simulink library "MonoDetector"  (R2022b)
settings: Solver=VariableStepAuto  StartTime=0.0  StopTime=10.0  RelTol=1e-3
undefined symbols (not defined in the file or in its folder): Row
libraries: TuneVar x14, TOP x12, StateVar x3, HandyTextFile x2, CapturedConstLib x2, FeaturePath x1, AudioStats x1, simulink x1, PoolIir x1
settings Model: Creator=ud1041536  LastModifiedBy=sc48041
settings SolverCC: AlgebraicLoopSolver=TrustRegion
settings DebuggingCC: UnconnectedInputMsg=warning  UnconnectedOutputMsg=warning  UnconnectedLineMsg=warning  SFMachineParentedDataDiag=warning  ArithmeticOperatorsInVariantConditions=warning
settings ModelReferenceCC: EnableRefExpFcnMdlSchedulingChecks=on
settings SFSimCC: CustomCodeUndefinedFunction=UseInterfaceOnly

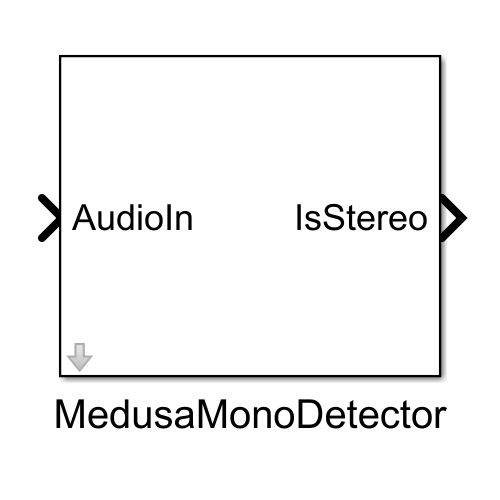
[thumbnail: Simulink's stored preview of the top-level diagram]
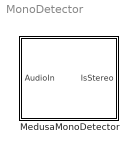
== system MonoDetector ==
  MedusaMonoDetector : Subsystem  mask(Mono Detector){Config=[]}
      mask prompts: Config "MedusaMonoDetectorConfig"
      mask help:
      | This block detects if given stereo input (L, R) is stereo. The output isStereo is used to enable/disable Spatial Unmasker in Medusa system. When the block is put to passthrough by tuning, the default output is set to 'true'.
      |
      | Configuration struct needs to define the below fields with the exact names which are used inside the block.
      |
      | decimationFactor: decimation factor
      | maxZeroLevelCount: maximum number of zero signals in a row before reset
      | hpfOrder: order of highpass filter
      | maxNumStages: maximum of sos for both L and R highpass filter
      | numChannels: number of channels
      |
      | For more information and sample generation of config struct, please see 'Help'.
      mask init:
      | blkh=gcbh;
      | Config=BTConfig.Assert(blkh,Config);
      | 
      | Config.Validate();
      mask Help:
      | Model that uses Mono Detector block need to call MonoDetectorInit(config) to generate <i>MonoDetectorConfigStruct</i> and <i>MonoDetectorTunable</i> bus object in base workspace.
      | 
      | <b>Sample usage:</b>
      | 
      | MedusaConfig = generateMedusaConfig(auto_gen_sys_defs);
      | MonoDetectorInit(MedusaConfig);
      | or
      | DefaultMedusaConfig = generateMedusaConfig();
      | MonoDetectorInit(DefaultMedusaConfig);

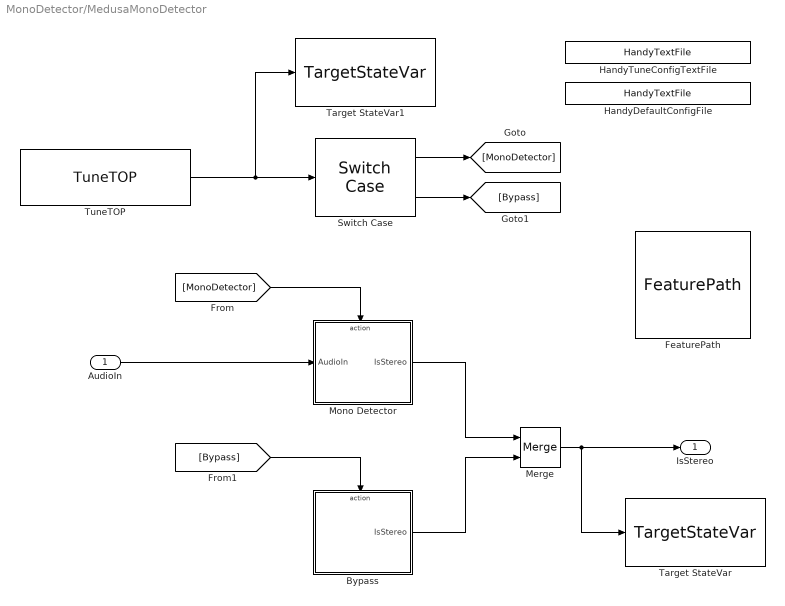
== system MonoDetector/MedusaMonoDetector ==
  AudioIn : Inport
  Bypass : Subsystem
  FeaturePath : FeaturePath/FeaturePath  FeatureName=MonoDetector  IsGroup=off  GroupNumber=-1  IsModule=off  TriggerInit=[680 129 795 236]
      settings: SourceProductName=Bose Talaria
  HandyDefaultConfigFile : HandyTextFile/HandyTextFile  TemplateSource=Config  FileSuffix=Init  OpenDialogOnLoad=off  UseThisBlockName=off  AddGrandParentNamePrefix=off  TheDefaultText=|  ShowInLibBrowser=on
      | % $(FILENAME) Setup model parameters for each "Init" callback (e.g. update diagram)
      | sample_rate_in_hertz = 44100;
      | frame_size = 32;
      | sysin_channel_count = 2;
      settings: SourceProductName=Bose Talaria
  HandyTuneConfigTextFile : HandyTextFile/HandyTextFile  TemplateSource=TuneConfig  FileSuffix=Init  OpenDialogOnLoad=off  UseThisBlockName=off  AddGrandParentNamePrefix=off  TheDefaultText=|  ShowInLibBrowser=on
      | % $(FILENAME) Setup model parameters for each "Init" callback (e.g. update diagram)
      | sample_rate_in_hertz = 44100;
      | frame_size = 32;
      | sysin_channel_count = 2;
      settings: SourceProductName=Bose Talaria
  Merge : Merge
  Mono Detector : Subsystem
  Switch Case : SwitchCase
  Target StateVar : StateVar/TargetStateVar  TriggerInit=[670 396 810 464]  TspName=IsStereo  StateName=IsStereo  UseSameName=on  IfdefMacro=[]
      settings: SourceProductName=Bose Talaria
  Target StateVar1 : StateVar/TargetStateVar  TriggerInit=[340 131 480 199]  TspName=IsActive  StateName=IsActive  UseSameName=on  IfdefMacro=[]
      settings: SourceProductName=Bose Talaria
  TuneTOP : TuneVar/TuneTOP  TriggerInit=[65 47 235 103]  TopName=Enable  TuneName=Enable  DataTypeOut=int32  TunabilityNumber=1  MinValue=[]  MaxValue=[]  BankNumber=0  PreOverlay=false  PostOverlay=false  UseSameName=on  MaskValue=Config.TuneDefaults.Enable
      settings: SourceProductName=Bose Talaria
  IsStereo : Outport  VectorParamsAs1DForOutWhenUnconnected=off
  wires:
  Merge/1 -> Target StateVar/1, IsStereo/1
  Switch Case/1 -> [MonoDetector]
  TuneTOP/1 -> Switch Case/1, Target StateVar1/1
  AudioIn/1 -> Mono Detector/1(AudioIn)
  Bypass/1(IsStereo) -> Merge/2
  Switch Case/2 -> [Bypass]
  Mono Detector/1(IsStereo) -> Merge/1
  [Bypass] -> Bypass/Action
  [MonoDetector] -> Mono Detector/Action

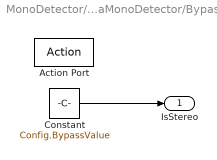
== system MonoDetector/MedusaMonoDetector/Bypass ==
  Action Port : ActionPort  ActionPortLabel=default: { }
  Constant : Constant  Value=Config.BypassValue  OutDataTypeStr=uint32
  IsStereo : Outport  VectorParamsAs1DForOutWhenUnconnected=off
  wires:
  Constant/1 -> IsStereo/1

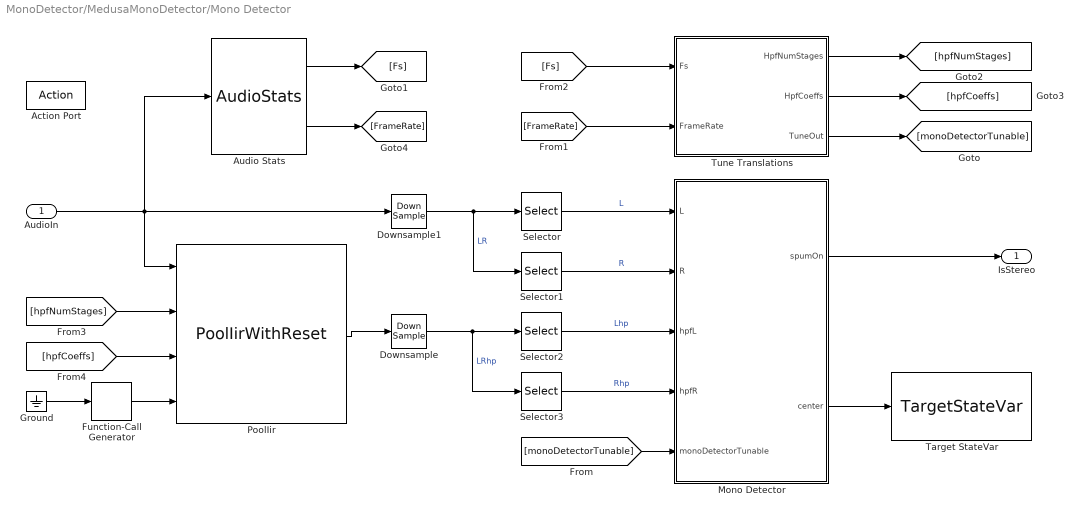
== system MonoDetector/MedusaMonoDetector/Mono Detector ==
  AudioIn : Inport  OutDataTypeStr=single
  Action Port : ActionPort  ActionPortLabel=case: { }
  Audio Stats : AudioStats/AudioStats  DoSampleRate=on  TypeSampleRate=double  DoCallRate=on  TypeCallRate=double  DoFrameSize=off  TypeFrameSize=Inherit: auto  DoChannelCount=off  TypeChannelCount=Inherit: auto  DoTaskRateFactor=off  TypeTaskRateFactor=Inherit: auto  MacroNameRoot=AUDIO  MacroNameRootEval='AUDIO'  IsMacroNameEval=off  MacroSampleRate=off  MacroCallRate=off  MacroFrameSize=off  MacroChannelCount=off  MacroTaskRateFactor=off  MacroTaskId=off  ValidateSampleRate=off  ValueSampleRate=[]  ValidateCallRate=off  ValueCallRate=[]  ValidateFrameSize=off  ValueFrameSize=[]  ValidateChannelCount=off  ValueChannelCount=[]  ValidateTaskRateFactor=off  ValueTaskRateFactor=[]
      settings: SourceProductName=Bose Talaria
  Downsample : DownSample  N=Config.DownSamplingFactor
  Downsample1 : DownSample  N=Config.DownSamplingFactor
  Function-Call Generator : simulink/Ports & Subsystems/Function-Call Generator  sample_time=1  numberOfIterations=1  DisallowWideOutput=off  ShowEnablePort=on
  Ground : Ground
  Mono Detector : MATLAB Function  TreatAsAtomicUnit=on  mask{maxZeroLevelCount=Config.MaxZeroLevelCount}
  PoolIir : PoolIir/PoolIirWithReset  Config=Config.Hpf
  Selector : Selector  InputPortWidth=2  IndexOptions=Index vector (dialog)  Indices=1  OutputSizes=1
  Selector1 : Selector  InputPortWidth=2  IndexOptions=Index vector (dialog)  Indices=2  OutputSizes=1
  Selector2 : Selector  InputPortWidth=2  IndexOptions=Index vector (dialog)  Indices=1  OutputSizes=1
  Selector3 : Selector  InputPortWidth=2  IndexOptions=Index vector (dialog)  Indices=2  OutputSizes=1
  Target StateVar : StateVar/TargetStateVar  TriggerInit=[875 1951 1015 2019]  TspName=LevelCenter  StateName=LevelCenter  UseSameName=on  IfdefMacro=[]
      settings: SourceProductName=Bose Talaria
  Tune Translations : Subsystem
  IsStereo : Outport  VectorParamsAs1DForOutWhenUnconnected=off
  wires:
  Downsample1/1 -> Selector1/1, Selector/1  "LR"
  Mono Detector/2(center) -> Target StateVar/1
  Downsample/1 -> Selector3/1, Selector2/1  "LRhp"
  Selector/1 -> Mono Detector/1(L)  "L"
  [hpfCoeffs] -> PoolIir/3
  PoolIir/1 -> Downsample/1
  [hpfNumStages] -> PoolIir/2
  Selector1/1 -> Mono Detector/2(R)  "R"
  Audio Stats/1 -> [Fs]
  Mono Detector/1(spumOn) -> IsStereo/1
  [monoDetectorTunable] -> Mono Detector/5(monoDetectorTunable)
  Selector2/1 -> Mono Detector/3(hpfL)  "Lhp"
  Selector3/1 -> Mono Detector/4(hpfR)  "Rhp"
  AudioIn/1 -> PoolIir/1, Downsample1/1, Audio Stats/1
  Audio Stats/2 -> [FrameRate]
  [Fs] -> Tune Translations/1(Fs)
  [FrameRate] -> Tune Translations/2(FrameRate)
  Tune Translations/3(TuneOut) -> [monoDetectorTunable]
  Tune Translations/2(HpfCoeffs) -> [hpfCoeffs]
  Tune Translations/1(HpfNumStages) -> [hpfNumStages]
  Ground/1 -> Function-Call Generator/1
  Function-Call Generator/1 -> PoolIir/4

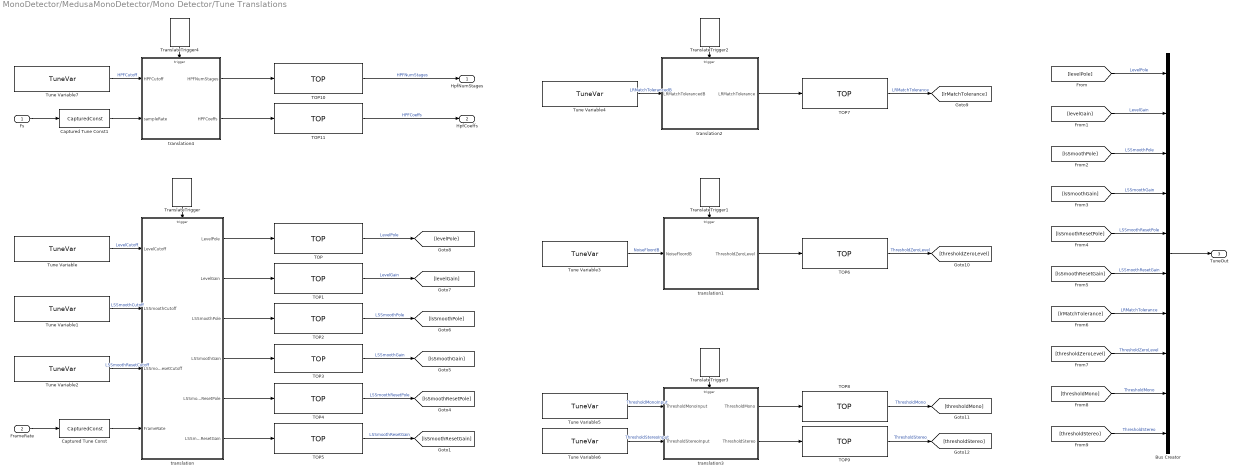
== system MonoDetector/MedusaMonoDetector/Mono Detector/Tune Translations ==
  Fs : Inport
  FrameRate : Inport  Port=2
  Bus Creator : BusCreator  Inputs=10  OutDataTypeStr=Bus: MonoDetectorTunable
      settings: InheritFromInputs=off
  Captured Tune Const : CapturedConstLib/CapturedConst  TriggerInit=[-1540 1092 -1440 1128]  Role=Automatic
      settings: SourceProductName=Bose Talaria
  Captured Tune Const1 : CapturedConstLib/CapturedConst  TriggerInit=[-1540 472 -1440 508]  Role=Automatic
      settings: SourceProductName=Bose Talaria
  TOP : TOP/TOP  TriggerInit=[-1110 700 -935 760]  TopName=LevelPole  DataTypeOut=single  BankNumber=0  PreOverlay=false  PostOverlay=false  Role=Automatic
      settings: SourceProductName=Bose Talaria
  TOP1 : TOP/TOP  TriggerInit=[-1110 780 -935 840]  TopName=LevelGain  DataTypeOut=single  BankNumber=0  PreOverlay=false  PostOverlay=false  Role=Automatic
      settings: SourceProductName=Bose Talaria
  TOP10 : TOP/TOP  TriggerInit=[-1110 380 -935 440]  TopName=HPFNumStages  DataTypeOut=uint32  BankNumber=0  PreOverlay=false  PostOverlay=false  Role=Automatic
      settings: SourceProductName=Bose Talaria
  TOP11 : TOP/TOP  TriggerInit=[-1110 460 -935 520]  TopName=HPFCoeffs  DataTypeOut=single  BankNumber=0  PreOverlay=false  PostOverlay=false  Role=Automatic
      settings: SourceProductName=Bose Talaria
  TOP2 : TOP/TOP  TriggerInit=[-1110 860 -935 920]  TopName=LSSmoothPole  DataTypeOut=single  BankNumber=0  PreOverlay=false  PostOverlay=false  Role=Automatic
      settings: SourceProductName=Bose Talaria
  TOP3 : TOP/TOP  TriggerInit=[-1110 942 -935 998]  TopName=LSSmoothGain  DataTypeOut=single  BankNumber=0  PreOverlay=false  PostOverlay=false  Role=Automatic
      settings: SourceProductName=Bose Talaria
  TOP4 : TOP/TOP  TriggerInit=[-1110 1020 -935 1080]  TopName=LSSmoothResetPole  DataTypeOut=single  BankNumber=0  PreOverlay=false  PostOverlay=false  Role=Automatic
      settings: SourceProductName=Bose Talaria
  TOP5 : TOP/TOP  TriggerInit=[-1110 1100 -935 1160]  TopName=LSSmoothResetGain  DataTypeOut=single  BankNumber=0  PreOverlay=false  PostOverlay=false  Role=Automatic
      settings: SourceProductName=Bose Talaria
  TOP6 : TOP/TOP  TriggerInit=[-55 730 115 790]  TopName=ThresholdZeroLevel  DataTypeOut=single  BankNumber=0  PreOverlay=false  PostOverlay=false  Role=Automatic
      settings: SourceProductName=Bose Talaria
  TOP7 : TOP/TOP  TriggerInit=[-55 410 115 470]  TopName=LRMatchTolerance  DataTypeOut=single  BankNumber=0  PreOverlay=false  PostOverlay=false  Role=Automatic
      settings: SourceProductName=Bose Talaria
  TOP8 : TOP/TOP  TriggerInit=[-55 1035 115 1095]  TopName=ThresholdMono  DataTypeOut=single  BankNumber=0  PreOverlay=false  PostOverlay=false  Role=Automatic
      settings: SourceProductName=Bose Talaria
  TOP9 : TOP/TOP  TriggerInit=[-55 1105 115 1165]  TopName=ThresholdStereo  DataTypeOut=single  BankNumber=0  PreOverlay=false  PostOverlay=false  Role=Automatic
      settings: SourceProductName=Bose Talaria
  TranslateTrigger : TuneVar/TranslateTrigger  TriggerInit=[-1314 610 -1276 665]
      settings: SourceProductName=Bose Talaria
  TranslateTrigger1 : TuneVar/TranslateTrigger  TriggerInit=[-259 610 -221 665]
      settings: SourceProductName=Bose Talaria
  TranslateTrigger2 : TuneVar/TranslateTrigger  TriggerInit=[-259 290 -221 345]
      settings: SourceProductName=Bose Talaria
  TranslateTrigger3 : TuneVar/TranslateTrigger  TriggerInit=[-259 950 -221 1005]
      settings: SourceProductName=Bose Talaria
  TranslateTrigger4 : TuneVar/TranslateTrigger  TriggerInit=[-1319 290 -1281 345]
      settings: SourceProductName=Bose Talaria
  Tune Variable : TuneVar/TuneVar  TuneName=LevelCutoff  SpecifyMaxSize=off  VariableDim=1 (Row)  MaxSize=[1 1]  TunabilityNumber=1  MinValue=[]  MaxValue=[]  TriggerInit=[-1630 725 -1440 775]  MaskValue=Config.TuneDefaults.LevelCutoff
      settings: SourceProductName=Bose Talaria
  Tune Variable1 : TuneVar/TuneVar  TuneName=LSSmoothCutoff  SpecifyMaxSize=off  VariableDim=1 (Row)  MaxSize=[1 1]  TunabilityNumber=1  MinValue=[]  MaxValue=[]  TriggerInit=[-1630 845 -1440 895]  MaskValue=Config.TuneDefaults.LSSmoothCutoff
      settings: SourceProductName=Bose Talaria
  Tune Variable2 : TuneVar/TuneVar  TuneName=LSSmoothResetCutoff  SpecifyMaxSize=off  VariableDim=1 (Row)  MaxSize=[1 1]  TunabilityNumber=1  MinValue=[]  MaxValue=[]  TriggerInit=[-1630 965 -1440 1015]  MaskValue=Config.TuneDefaults.LSSmoothResetCutoff
      settings: SourceProductName=Bose Talaria
  Tune Variable3 : TuneVar/TuneVar  TuneName=NoiseFloordB  SpecifyMaxSize=off  VariableDim=1 (Row)  MaxSize=[1 1]  TunabilityNumber=1  MinValue=[]  MaxValue=[]  TriggerInit=[-575 735 -405 785]  MaskValue=Config.TuneDefaults.NoiseFloordB
      settings: SourceProductName=Bose Talaria
  Tune Variable4 : TuneVar/TuneVar  TuneName=LRMatchTolerancedB  SpecifyMaxSize=off  VariableDim=1 (Row)  MaxSize=[1 1]  TunabilityNumber=1  MinValue=[]  MaxValue=[]  TriggerInit=[-575 415 -385 465]  MaskValue=Config.TuneDefaults.LRMatchTolerancedB
      settings: SourceProductName=Bose Talaria
  Tune Variable5 : TuneVar/TuneVar  TuneName=ThresholdMonoInput  SpecifyMaxSize=off  VariableDim=1 (Row)  MaxSize=[1 1]  TunabilityNumber=1  MinValue=[]  MaxValue=[]  TriggerInit=[-575 1040 -405 1090]  MaskValue=Config.TuneDefaults.ThresholdMonoInput
      settings: SourceProductName=Bose Talaria
  Tune Variable6 : TuneVar/TuneVar  TuneName=ThresholdStereoInput  SpecifyMaxSize=off  VariableDim=1 (Row)  MaxSize=[1 1]  TunabilityNumber=1  MinValue=[]  MaxValue=[]  TriggerInit=[-575 1110 -405 1160]  MaskValue=Config.TuneDefaults.ThresholdStereoInput
      settings: SourceProductName=Bose Talaria
  Tune Variable7 : TuneVar/TuneVar  TuneName=HPFCutoff  SpecifyMaxSize=off  VariableDim=1 (Row)  MaxSize=[1 1]  TunabilityNumber=1  MinValue=[]  MaxValue=[]  TriggerInit=[-1630 385 -1440 435]  MaskValue=Config.TuneDefaults.HPFCutoff
      settings: SourceProductName=Bose Talaria
  translation : MATLAB Function  TreatAsAtomicUnit=on
  translation1 : MATLAB Function  TreatAsAtomicUnit=on
  translation2 : MATLAB Function  TreatAsAtomicUnit=on
  translation3 : MATLAB Function  TreatAsAtomicUnit=on
  translation4 : MATLAB Function  TreatAsAtomicUnit=on  mask{numChannels=Config.NumInputChannels, maxNumStages=Config.Hpf.MaxNumStages}
  HpfNumStages : Outport
  HpfCoeffs : Outport  Port=2
  TuneOut : Outport  Port=3
  wires:
  Tune Variable1/1 -> translation/2(LSSmoothCutoff)  "LSSmoothCutoff"
  Tune Variable6/1 -> translation3/2(ThresholdStereoInput)  "ThresholdStereoInput"
  translation3/1(ThresholdMono) -> TOP8/1
  [thresholdMono] -> Bus Creator/9  "ThresholdMono"
  [lsSmoothResetGain] -> Bus Creator/6  "LSSmoothResetGain"
  Tune Variable/1 -> translation/1(LevelCutoff)  "LevelCutoff"
  [lsSmoothResetPole] -> Bus Creator/5  "LSSmoothResetPole"
  Tune Variable4/1 -> translation2/1(LRMatchTolerancedB)  "LRMatchTolerancedB"
  translation/3(LSSmoothPole) -> TOP2/1
  translation4/2(HPFCoeffs) -> TOP11/1
  translation/5(LSSmoothResetPole) -> TOP4/1
  FrameRate/1 -> Captured Tune Const/1
  TOP10/1 -> HpfNumStages/1  "HPFNumStages"
  [thresholdZeroLevel] -> Bus Creator/8  "ThresholdZeroLevel"
  Captured Tune Const/1 -> translation/4(FrameRate)
  TranslateTrigger2/1 -> translation2/Trigger
  translation3/2(ThresholdStereo) -> TOP9/1
  TranslateTrigger3/1 -> translation3/Trigger
  [thresholdStereo] -> Bus Creator/10  "ThresholdStereo"
  TranslateTrigger1/1 -> translation1/Trigger
  Tune Variable5/1 -> translation3/1(ThresholdMonoInput)  "ThresholdMonoInput"
  Tune Variable7/1 -> translation4/1(HPFCutoff)  "HPFCutoff"
  translation2/1(LRMatchTolerance) -> TOP7/1
  Fs/1 -> Captured Tune Const1/1
  translation/4(LSSmoothGain) -> TOP3/1
  Bus Creator/1 -> TuneOut/1
  [lrMatchTolerance] -> Bus Creator/7  "LRMatchTolerance"
  TranslateTrigger4/1 -> translation4/Trigger
  TranslateTrigger/1 -> translation/Trigger
  [levelPole] -> Bus Creator/1  "LevelPole"
  translation1/1(ThresholdZeroLevel) -> TOP6/1
  TOP11/1 -> HpfCoeffs/1  "HPFCoeffs"
  [levelGain] -> Bus Creator/2  "LevelGain"
  [lsSmoothGain] -> Bus Creator/4  "LSSmoothGain"
  Captured Tune Const1/1 -> translation4/2(sampleRate)
  Tune Variable3/1 -> translation1/1(NoiseFloordB)  "NoiseFloordB"
  translation/6(LSSmoothResetGain) -> TOP5/1
  translation4/1(HPFNumStages) -> TOP10/1
  translation/1(LevelPole) -> TOP/1
  Tune Variable2/1 -> translation/3(LSSmoothResetCutoff)  "LSSmoothResetCutoff"
  translation/2(LevelGain) -> TOP1/1
  [lsSmoothPole] -> Bus Creator/3  "LSSmoothPole"
  TOP5/1 -> [lsSmoothResetGain]  "LSSmoothResetGain"
  TOP4/1 -> [lsSmoothResetPole]  "LSSmoothResetPole"
  TOP3/1 -> [lsSmoothGain]  "LSSmoothGain"
  TOP2/1 -> [lsSmoothPole]  "LSSmoothPole"
  TOP1/1 -> [levelGain]  "LevelGain"
  TOP/1 -> [levelPole]  "LevelPole"
  TOP7/1 -> [lrMatchTolerance]  "LRMatchTolerance"
  TOP6/1 -> [thresholdZeroLevel]  "ThresholdZeroLevel"
  TOP8/1 -> [thresholdMono]  "ThresholdMono"
  TOP9/1 -> [thresholdStereo]  "ThresholdStereo"

== matlab function MonoDetector/MedusaMonoDetector/Mono Detector/Tune Translations/translation1 ==
  data: ThresholdZeroLevel output; NoiseFloordB input
  events: trigger input FUNCTION_CALL_EVENT
function ThresholdZeroLevel  = fcn(NoiseFloordB)
% thresh = 2 * undb20(noiseFloordB)
ThresholdZeroLevel = 2 * (10 ^ (NoiseFloordB.Value / 20));

== matlab function MonoDetector/MedusaMonoDetector/Mono Detector/Mono Detector ==
  data: L input; spumOn output; R input; hpfL input; hpfR input; center output; monoDetectorTunable input; maxZeroLevelCount parameter
function [spumOn, center]  = monoDetect(L, R, hpfL, hpfR, ...
                                monoDetectorTunable, maxZeroLevelCount)
%#codegen

persistent zeroLevelCount;
persistent Llevel;
persistent Rlevel;
persistent smoothedSumOfEnergies;
persistent smoothedEnergyOfSum;
persistent levelCenter;
persistent lastSpumOn; % basically isStereo, since we turn on SPUM if input is stereo

if isempty(zeroLevelCount); zeroLevelCount = 0; end
if isempty(Llevel); Llevel = single(0); end
if isempty(Rlevel); Rlevel = single(0); end
if isempty(smoothedSumOfEnergies); smoothedSumOfEnergies = single(0); end
if isempty(smoothedEnergyOfSum); smoothedEnergyOfSum = single(0); end
if isempty(levelCenter); levelCenter = single(0); end
if isempty(lastSpumOn); lastSpumOn = true; end

absLeft = abs(L);
absRight = abs(R);

% Recursive averaging
a1 = monoDetectorTunable.levelPole;
b0 = monoDetectorTunable.levelGain;
Llevel = Llevel * a1 +  absLeft * b0;
Rlevel = Rlevel * a1 +  absRight * b0;

% Compute saturated signals from predetermined miss-match tolerance
LlevelSat = min(Llevel, Rlevel*monoDetectorTunable.leftRightMatchTolerance);
RlevelSat = min(Rlevel, Llevel*monoDetectorTunable.leftRightMatchTolerance);

% Compute mono content variables
curL = hpfL * RlevelSat;
curR = hpfR * LlevelSat;
sumOfEnergies = curL^2 + curR^2; % tgtX2
energyOfSum = 0.5*(curL + curR)^2; % tgtX2Center

% Check if signal has been low for awhile
if (absLeft + absRight) < monoDetectorTunable.thresholdZeroLevel
    zeroLevelCount = zeroLevelCount + 1;
else 
    zeroLevelCount = 0;
end

% Pole selection (determine LPF coefficient) for least square smoothing
% If the signal level is very low (or zero) for awhile, rest params and 
% select correct poles so that we don't miss fast changes in input
if zeroLevelCount > maxZeroLevelCount
    sumOfEnergies = single(0);
    energyOfSum = single(0);
    smoothedSumOfEnergies = single(0);
    smoothedEnergyOfSum = single(0);
    lsPole = monoDetectorTunable.lsSmoothResetPole;
    lsGain = monoDetectorTunable.lsSmoothResetGain;
    zeroLevelCount = maxZeroLevelCount + 1;
else
    lsPole = monoDetectorTunable.lsSmoothPole;
    lsGain = monoDetectorTunable.lsSmoothGain;
end

% Least square smoothing 
smoothedSumOfEnergies = lsPole * smoothedSumOfEnergies + lsGain * sumOfEnergies;
smoothedEnergyOfSum = lsPole * smoothedEnergyOfSum + lsGain * energyOfSum;

% Compute measure of center (or mono) level
levelCenter = smoothedEnergyOfSum/(smoothedSumOfEnergies + single(eps));

% Determine if input is stereo and turn SPUM on/off accordingly
% stereo case 1: was stereo last time (SPUM on) and this mono level < mono threhold
% stereo case 2: was mono last time (SPUM off) and this mono level < stereo threshold
lastSpumOn = (lastSpumOn && (levelCenter < monoDetectorTunable.thresholdMono)) ...
    || (~lastSpumOn && (levelCenter <= monoDetectorTunable.thresholdStereo));

spumOn = uint32(lastSpumOn);% equivalent to isStereo

center = levelCenter;

end

== matlab function MonoDetector/MedusaMonoDetector/Mono Detector/Tune Translations/translation2 ==
  data: LRMatchTolerance output; LRMatchTolerancedB input
  events: trigger input FUNCTION_CALL_EVENT
function LRMatchTolerance  = fcn(LRMatchTolerancedB)

if (LRMatchTolerancedB.Value < 0 || LRMatchTolerancedB.Value > 0.5)
    TranslateError('Invalid tolerance for left right match');
    LRMatchTolerance = 0;
else
    LRMatchTolerance = 10 ^ (LRMatchTolerancedB.Value / 20);
end

== matlab function MonoDetector/MedusaMonoDetector/Mono Detector/Tune Translations/translation3 ==
  data: ThresholdMono output; ThresholdMonoInput input; ThresholdStereoInput input; ThresholdStereo output
  events: trigger input FUNCTION_CALL_EVENT
function [ThresholdMono, ThresholdStereo] = fcn(ThresholdMonoInput, ThresholdStereoInput)
% The exponent 1/64 is carried over from AR and old bdsp implementation.
% This is designed by Chris Cheng to make the gap between two thresholds
% as small as possible, because in theory they should be almost identical.
% Removing this would still work in theory with a slight change in the 
% output. However as we verify the block against PREQ Simulink model, this
% translation is retained to get a complete match in performance.

if ThresholdMonoInput.Value <= ThresholdStereoInput.Value
    TranslateError('Threshold for mono should be higher than that for stereo');
    ThresholdMono = 0;
    ThresholdStereo = 0;
elseif (ThresholdMonoInput.Value >= 1) || (ThresholdStereoInput.Value >= 1)
    TranslateError('Threshold values for mono and stereo should be less than 1.0');
    ThresholdMono = 0;
    ThresholdStereo = 0;
else
    ThresholdMono = ThresholdMonoInput.Value ^ (1/64);
    ThresholdStereo = ThresholdStereoInput.Value ^ (1/64);
end

== matlab function MonoDetector/MedusaMonoDetector/Mono Detector/Tune Translations/translation4 ==
  data: HPFNumStages output; HPFCutoff input; sampleRate input; HPFCoeffs output; numChannels parameter; maxNumStages parameter
  events: trigger input FUNCTION_CALL_EVENT
function [HPFNumStages, HPFCoeffs] = fcn(HPFCutoff, sampleRate, numChannels, maxNumStages)
%#codegen
%[Param:numChannels]
%[Param:maxNumStages]

% Calculation is fixed for a second order high pass butterworth, i.e. this 
% translation will not work anymore if the filter order/design is changed. 
% Code for computing hpf is taken from AR model.
% More generic implementation is also included below. In this case of 2nd 
% order filter, we get better precision by getting the one-stage sos 
% directly from the transfer function.

% hpfOrder = configStruct.hpfOrder;
% normFreq = 2 * HPFCutoff.Value / sampleRate;
% [Z, P, K] = butter_for_code_gen(hpfOrder, hpfOrder, normFreq, 'high');
% sos = zp2sos_for_code_gen(Z, P, K);

w = 2 * pi* HPFCutoff.Value / sampleRate;
sqrt2 = sqrt(2);
sinw = sin(w);
cosw = cos(w);

if (HPFCutoff.Value <= 0) || (HPFCutoff.Value > sampleRate/2)
    TranslateError('Highpass filter cutoff is out of range; should be in (0, %d)',sampleRate/2);
    b = single([1 0 0]);
    a = single([1 0 0]);
else
    denom = (sqrt2 + sinw);
    a1 = -2 * sqrt2 * cosw / denom;
    a2 = (sqrt2 - sinw) / denom;
    a = single([1 a1 a2]);
    b = single([1 -2 1] * (1-a1+a2) / 4);
end
sos = [b,a];

numStages = size(sos, 1) * ones(1, numChannels);
rawSOS = repmat(sos, numChannels, 1);

[HPFNumStages, HPFCoeffs] = pooliirTranslation(rawSOS, numStages, maxNumStages);

end


function [PoolNumStages, PoolCoeffs] = pooliirTranslation(rawSOS, numStages, maxNumStages)
% Function to format sos into pooliir. Taken from Translation block
% inside pooliir library block.

RawSOS = rawSOS;
NumStages = int32(numStages);
NumChannels = length(NumStages);

MaxNumStages = maxNumStages; 
PoolNumStages = int32(zeros(NumChannels,1));
PoolCoeffs = double(zeros(MaxNumStages * 4 + NumChannels,1));
ChannelCoeffs = zeros(MaxNumStages * 4 + 1,1);
ChannelSOS = double(zeros(MaxNumStages, 6));
SOSIndex = int32(0);

for i = 1:NumChannels
    
    ChannelNumStages = NumStages(i);   % Size of current SOS
    assert(ChannelNumStages <= MaxNumStages);
    
    ChannelSOS(1:ChannelNumStages,:) = RawSOS(SOSIndex+(1:ChannelNumStages),:);
    SOSIndex = SOSIndex + ChannelNumStages;

    if size(ChannelSOS,2) ~= 6
        TranslateError('SOS matrix must have 6 columns');
    end
    % decompose SOS
   
    ts = 1:4:4*ChannelNumStages;
    ChannelCoeffs(1,1) = prod(ChannelSOS(1:ChannelNumStages,1));        % b0
    
    % the remaining coeffs are compacted forms of the biquads
    ChannelCoeffs(1+ts,1) = ChannelSOS(1:ChannelNumStages,6);           % a2
    ChannelCoeffs(2+ts,1) = ChannelSOS(1:ChannelNumStages,5);           % a1
    if( ChannelSOS(:,1) == 0 )
    ChannelCoeffs(3+ts,1) = 0;                 % b2/b0
    ChannelCoeffs(4+ts,1) = 0;                 % b1/b0
    else
    ChannelCoeffs(3+ts,1) = ...
        ChannelSOS(1:ChannelNumStages,3)./ ...
        ChannelSOS(1:ChannelNumStages,1);  % b2/b0
    ChannelCoeffs(4+ts,1) = ...
        ChannelSOS(1:ChannelNumStages,2)./ ...
        ChannelSOS(1:ChannelNumStages,1);  % b1/b0
    end
    
    % length of Current Channel Coeffs
    ChannelCoeffsLength = 1+4*ChannelNumStages;
    
    % Offset into coefficient array for the current channel
    offset = (i-1)+4*sum(PoolNumStages(1:i-1));
    
    % Verify that the SOS does not violate the maximum number of stages
    % allocated for the pool
    PoolNumStages(i) = int32(ChannelNumStages);
    if sum(PoolNumStages) > MaxNumStages
        TranslateError('Too many second order sections');
    end

    % Store the coefficients
    PoolCoeffs(offset+(1:ChannelCoeffsLength)) = double(ChannelCoeffs(1:ChannelCoeffsLength));   
end
end

== matlab function MonoDetector/MedusaMonoDetector/Mono Detector/Tune Translations/translation ==
  data: LevelPole output; LevelCutoff input; LevelGain output; LSSmoothCutoff input; LSSmoothResetCutoff input; LSSmoothPole output; LSSmoothGain output; LSSmoothResetPole output; LSSmoothResetGain output; FrameRate input
  events: trigger input FUNCTION_CALL_EVENT
function [LevelPole, LevelGain, LSSmoothPole, LSSmoothGain, ...
    LSSmoothResetPole, LSSmoothResetGain] = fcn(LevelCutoff, ...
    LSSmoothCutoff, LSSmoothResetCutoff, FrameRate)

% Cutoff is the inverse of time constant in Hz. So this function
% basically converts reciprocal of time constant to first order iir
% filter coefficient.
% Reference: https://bosecorp.sharepoint.com/sites/ASD3/DSPTeam/Shared%20Documents/DSP_Topics/Comparison%20of%20time%20constant%20conversion%20methods.docx

error = false;
if LevelCutoff.Value <= LSSmoothCutoff.Value
    TranslateError('Least square smoother should smooth more than level smoother');
    error = true;
elseif LSSmoothResetCutoff.Value <= LSSmoothCutoff.Value
    TranslateError('Least square smoother for reset should smooth less than that for normal mode');
    error = true;
end

if (~error)
    wn = 2 * pi * LevelCutoff.Value / FrameRate;
    LevelPole = (1 - sin(wn)) ./ cos(wn);
    LevelGain = 1 - LevelPole;

    wn = 2 * pi * LSSmoothCutoff.Value / FrameRate;
    LSSmoothPole = (1 - sin(wn)) ./ cos(wn);
    LSSmoothGain = 1 - LSSmoothPole;

    wn = 2 * pi * LSSmoothResetCutoff.Value / FrameRate;
    LSSmoothResetPole = (1 - sin(wn)) ./ cos(wn);
    LSSmoothResetGain = 1 - LSSmoothResetPole;
else
    LevelPole = 0;
    LevelGain = 0;
    LSSmoothPole = 0;
    LSSmoothGain = 0;   
    LSSmoothResetPole = 0;
    LSSmoothResetGain = 0;     
end

end
